simulink model "stem3d_2vehicles_v2011a_v2"  (Simulink 7.7)
settings: Solver=ode45  StartTime=0.0  StopTime=10.0  RelTol=1e-3
settings Model: Creator=LAPAN1  LastModifiedBy=LAPAN1
settings SolverCC: AutoInsertRateTranBlk=on
settings DataIOCC: SignalLoggingSaveFormat=Dataset
settings OptimizationCC: ExpressionDepthLimit=128
settings DebuggingCC: UnderspecifiedInitializationDetection=Simplified  FcnCallInpInsideContextMsg=Enable All  StateNameClashWarn=none
settings CodeAppCC: CustomSymbolStrType=$N$R$M_T
settings GRTTargetCC: TargetFunctionLibrary=C89/C90 (ANSI)

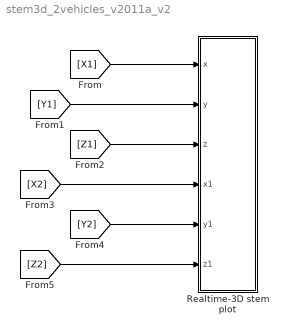
== system stem3d_2vehicles_v2011a_v2 ==
  Realtime-3D stem plot : Stateflow chart  TreatAsAtomicUnit=on
      settings: PermitHierarchicalResolution=ParametersOnly
  wires:
  [X1] -> Realtime-3D stem plot/1(x)
  [Y1] -> Realtime-3D stem plot/2(y)
  [Z1] -> Realtime-3D stem plot/3(z)
  [X2] -> Realtime-3D stem plot/4(x1)
  [Y2] -> Realtime-3D stem plot/5(y1)
  [Z2] -> Realtime-3D stem plot/6(z1)

== matlab function Realtime-3D stem plot ==
  data: x input double; y input double; z input double; x1 input double; y1 input double; z1 input double
function  fcn(x, y, z, x1, y1, z1)
figure(1);
hold on; grid on;
coder.extrinsic('stem3');
stem3(x, y, z, 'd', 'k' );
stem3(x1, y1, z1, '+', 'm' );

% coder.extrinsic('plot3');
% plot3(x, y, z, 'd', 'k' );
% plot3(x1, y1, z1, '+', 'm' );

view([45 45]);
